simulink model "quaternion_control_C3"  (R2016a)
settings: Solver=VariableStepAuto  StartTime=0.0  StopTime=10.0  RelTol=1e-3
undefined symbols (not defined in the file): tau_q
settings Model: Creator=mgreiff  LastModifiedBy=mgreiff

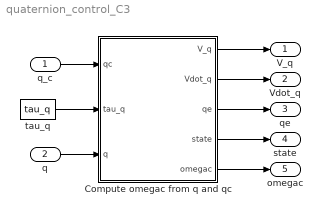
== system quaternion_control_C3 ==
  q_c : Inport  PortDimensions=4
  q : Inport  Port=2  PortDimensions=4
  Compute omegac from q and qc : MATLAB Function  TreatAsAtomicUnit=on
  tau_q : Constant  Value=tau_q
  V_q : Outport  PortDimensions=1
  Vdot_q : Outport  Port=2  PortDimensions=1
  qe : Outport  Port=3  PortDimensions=4
  state : Outport  Port=4  PortDimensions=1
  omegac : Outport  Port=5  PortDimensions=3
  wires:
  q_c/1 -> Compute omegac from q and qc/1(qc)
  q/1 -> Compute omegac from q and qc/3(q)
  tau_q/1 -> Compute omegac from q and qc/2(tau_q)
  Compute omegac from q and qc/1(V_q) -> V_q/1
  Compute omegac from q and qc/2(Vdot_q) -> Vdot_q/1
  Compute omegac from q and qc/3(qe) -> qe/1
  Compute omegac from q and qc/4(state) -> state/1
  Compute omegac from q and qc/5(omegac) -> omegac/1

== matlab function quaternion_control_C3/Compute omegac from q and qc ==
  data: V_q output; Vdot_q output; qe output; state output; qc input; tau_q input; q input; omegac output
function [V_q, Vdot_q, qe, state, omegac] = C3(qc, tau_q, q)
    % ~~~~~~~~~ Copyright (c) 2018 Marcus Greiff (see LICENCE.md) ~~~~~~~~~
    %
    % The hybrid quaternion-based control law for attitude control of the 
    % attitude dynamics.
    % 
    %     [V_q, Vdot_q, qe, state, omegac] = C3(qc, tau_q, q)
    % 
    % Here, qc is a commanded attitude, q is the measured or estimated
    % attitude and tau_q is a time-constant determining the rate of
    % convergence in the attitude controller. The outputs of the function
    % are as follows
    % 
    % V_q    - Lyapunov function in time
    % Vdot_q - Lyapunov function time derivative
    % qe     - Quaternion error measure on SO(4)
    % state  - The discrete state of the hybrid automata
    % omegac - The controlled attitude rate
    qc = qc./norm(qc);
    q = q./norm(q);
    
    qe = leftProduct(inverse(q))*qc;
    qi = [1;0;0;0];
    
    if qe(1) > 0
        V_q = (qe - qi)'*(qe - qi);
        state = 1;
    else
        V_q = (qe + qi)'*(qe + qi);
        state = -1;
    end
    Vdot_q = -(2/tau_q) * qe(2:4)'*qe(2:4);
    omegac = (2/tau_q) * sign(real(qe)) * imaginary(qe);
end

function S = skew(v)
    vx = v(1);
    vy = v(2);
    vz = v(3);
    S = [0 -vz vy; vz 0 -vx; -vy vx 0];
end

function qL = leftProduct(q)
    qw = q(1);
    qv = q(2:4);
    qL = qw*eye(4) + [0, -qv'; qv, skew(qv)];
end

function qinv = inverse(q)
    qinv=zeros(4,1);
    qinv(1) = q(1);
    qinv(2:4) = -q(2:4);
end

function qreal = real(q)
    qreal = q(1);
end

function qimaginary = imaginary(q)
    qimaginary = q(2:4);
end

function value = sign(v)
    if v >= 0
        value = 1;
    elseif v < 0
        value = -1;
    else
        value = 0;
    end
end
